simulink model "DFA"  (R2020a)
settings: Solver=VariableStepAuto  StartTime=0.0  StopTime=5  RelTol=1e-3
settings Model: Creator=none  LastModifiedBy=none

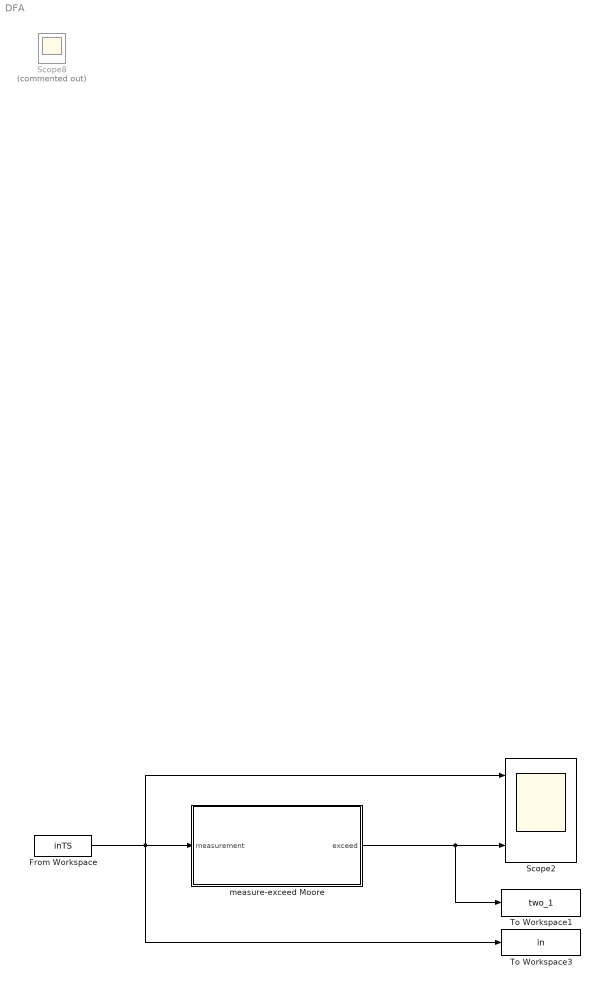
== system DFA ==
  From Workspace : FromWorkspace  VariableName=inTS  SampleTime=1
  Scope2 : Scope  NumInputPorts=3
  Scope8 : Scope  Commented=on  NumInputPorts=4
  To Workspace1 : ToWorkspace  VariableName=two_1  SaveFormat=Timeseries  SampleTime=-1
  To Workspace3 : ToWorkspace  VariableName=in  SaveFormat=Timeseries  SampleTime=-1
  measure-exceed Moore : Stateflow chart  TreatAsAtomicUnit=on
  wires:
  measure-exceed Moore/1(exceed) -> To Workspace1/1, Scope2/3
  From Workspace/1 -> To Workspace3/1, Scope2/1, measure-exceed Moore/1(measurement)

== stateflow chart DFA/measure-exceed Moore ==
  settings: stateMachineType=MOORE_MACHINE
  state Name
    exceed=0
  state Name1
    exceed=0
  state Name8
    exceed=1
  state Name2
    exceed=0
  state Name3
    exceed=0
  state Name4
    exceed=0
  state Name5
    exceed=0
  state Name6
    exceed=0
  state Name7
    exceed=0
  (default) -> Name
  Name1 -> Name8 [order 1] : [measurement==1]
  Name -> Name1 : [measurement==1]
  Name1 -> Name2 [order 2] : [measurement==0]
  Name5 -> Name8 [order 1] : [measurement==1]
  Name7 -> Name8 : [measurement==1]
  Name2 -> Name8 [order 2] : [measurement==1]
  Name6 -> Name8 [order 1] : [measurement==1]
  Name4 -> Name8 [order 2] : [measurement==1]
  Name3 -> Name8 [order 2] : [measurement==1]
  Name2 -> Name3 [order 1] : [measurement==0]
  Name3 -> Name4 [order 1] : [measurement==0]
  Name4 -> Name5 [order 1] : [measurement==0]
  Name5 -> Name6 [order 2] : [measurement==0]
  Name6 -> Name7 [order 2] : [measurement==0]
  data: measurement input; exceed output
